simulink model "Frist_ring_control_simulink"  (R2024b)
settings: Solver=VariableStepAuto  StartTime=0.0  StopTime=30  MaxStep=0.01  RelTol=1e-3
libraries: simulink x1
settings Model: Creator=DONGMO ZEWO  LastModifiedBy=DONGMO ZEWO

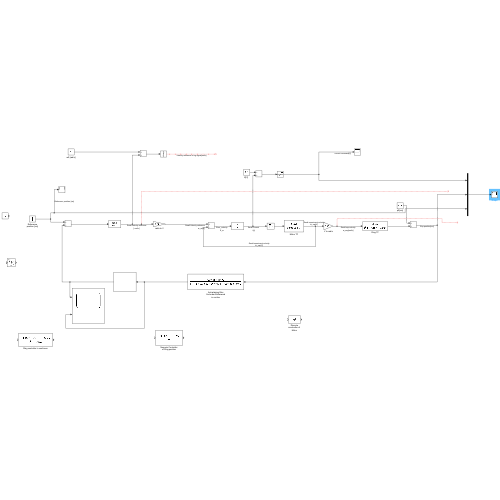
[thumbnail: Simulink's stored preview of the top-level diagram]
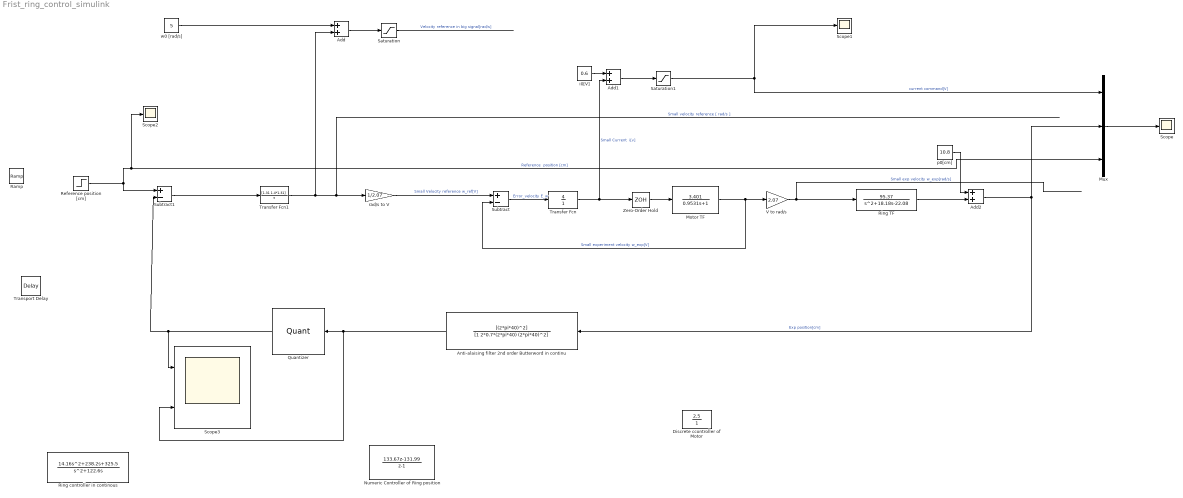
== system Frist_ring_control_simulink ==
  Add : Sum
  Add1 : Sum
  Add2 : Sum
  Anti-alaising filter 2nd order Butterword in continu : TransferFcn  Numerator=[(2*pi*40)^2]  Denominator=[1 2*0.7*(2*pi*40) (2*pi*40)^2]
  Discrete ccontroller of Motor : DiscreteTransferFcn  Numerator=[2.5]  Denominator=[1 ]
  Motor TF : TransferFcn  Numerator=[3.401]  Denominator=[0.9531 1]
  Mux : Mux  Inputs=3
  Numeric Controller of Ring position : DiscreteTransferFcn  Numerator=[133.67 -131.99]  Denominator=[1 -1]
  Quantizer : Quantizer  QuantizationInterval=1
  Ramp : simulink/Sources/Ramp  slope=0.84  start=0  InitialOutput=10.8
  Reference position [cm] : Step  Time=5  Before=10.8  After=13  SampleTime=0
  Ring TF : TransferFcn  Numerator=[95.37]  Denominator=[1 18.18 -22.08]
  Ring controller in continous : TransferFcn  Numerator=[14.16 238.2 325.5]  Denominator=[1 122.6 0]
  Saturation : Saturate
  Saturation1 : Saturate  UpperLimit=10  LowerLimit=-10
  Scope : Scope
  Scope1 : Scope
  Scope2 : Scope
  Scope3 : Scope  NumInputPorts=2
  Subtract : Sum  Inputs=+-
  Subtract1 : Sum  Inputs=+-
  Transfer Fcn : TransferFcn  Numerator=[4]  Denominator=[1]
  Transfer Fcn1 : TransferFcn  Numerator=[1.31 1.4*1.31]  Denominator=[1 0]
  Transport Delay : TransportDelay  DelayTime=0.01/2
  V to rad/s : Gain  Gain=2.07
  Zero-Order Hold : ZeroOrderHold  SampleTime=-1
  "i0[V]  " : Constant  Value=0.6
  p0[cm] : Constant  Value=10.8
  rad/s to V : Gain  Gain=1/2.07
  w0 [rad/s] : Constant  Value=5
  wires:
  Reference position [cm]/1 -> Subtract1/1, Mux/3, Scope2/1  "Reference  position [cm]"
  Subtract1/1 -> Transfer Fcn1/1
  Transfer Fcn1/1 -> rad/s to V/1, Add/2  "Small velocity reference [ rad/s ]"
  w0 [rad/s]/1 -> Add/1
  rad/s to V/1 -> Subtract/1  "Small Velocity reference w_ref[V]"
  Add/1 -> Saturation/1
  Subtract/1 -> Transfer Fcn/1  "Error_velocity E_w"
  Transfer Fcn/1 -> Zero-Order Hold/1, Add1/2  "Small Current  i[v]"
  "i0[V]  "/1 -> Add1/1
  Add1/1 -> Saturation1/1
  Motor TF/1 -> V to rad/s/1, Subtract/2  "Small experiment velocity w_exp[V]"
  p0[cm]/1 -> Add2/1
  Anti-alaising filter 2nd order Butterword in continu/1 -> Scope3/2, Quantizer/1
  Add2/1 -> Mux/2, Anti-alaising filter 2nd order Butterword in continu/1  "Exp position[cm]"
  Saturation1/1 -> Mux/1, Scope1/1  "current command[V]"
  V to rad/s/1 -> Ring TF/1  "Small exp velocity w_exp[rad/s]"
  Saturation/1 -> ?  "Velocity reference in big signal[rad/s]"
  Ring TF/1 -> Add2/2
  Zero-Order Hold/1 -> Motor TF/1
  Mux/1 -> Scope/1
  Quantizer/1 -> Scope3/1, Subtract1/2
